simulink model "rtwdemo_preprocessor"  (Simulink 7.6)
settings: Solver=FixedStepDiscrete  StartTime=0.0  StopTime=100  FixedStep=1  RelTol=1e-3
PostLoadFcn:
  | load rtwdemo_preprocessor_data.mat
Description:
  | Code Variants Using Model Blocks
settings Model: Creator=The MathWorks Inc.
settings DataIOCC: SaveFormat=StructureWithTime
settings OptimizationCC: InlineParams=on  InlineInvariantSignals=on  StrengthReduction=on  PassReuseOutputArgsAs=Individual arguments  ZeroExternalMemoryAtStartup=off  ZeroInternalMemoryAtStartup=off  OptimizeModelRefInitCode=on  LifeSpan=1
settings DebuggingCC: MergeDetectMultiDrivingBlocksExec=error  UniqueDataStoreMsg=error  ModelReferenceSymbolNameMessage=none  StrictBusMsg=ErrorOnBusTreatedAsVector
settings HardwareCC: ProdIntDivRoundTo=Zero  ProdEndianess=LittleEndian  ProdHWDeviceType=Generic->32-bit Embedded Processor
settings ModelReferenceCC: ModelReferencePassRootInputsByReference=off
settings RTWCC: SystemTargetFile=ert.tlc  TemplateMakefile=ert_default_tmf  Description=Real-Time Workshop Embedded Coder  GenerateReport=on  RTWVerbose=off  ProcessScript=ert_make_rtw_hook  IncludeHyperlinkInReport=on  LaunchReport=on
settings CodeAppCC: IgnoreCustomStorageClasses=off  IgnoreTestpoints=on
settings ERTTargetCC: MultiwordLength=2048  GenerateSampleERTMain=on  SupportNonFinite=off  InlinedParameterPlacement=NonHierarchical  ERTCustomFileTemplate=example_file_process.tlc  ERTFilePackagingFormat=CompactWithDataFile  ConvertIfToSwitch=off

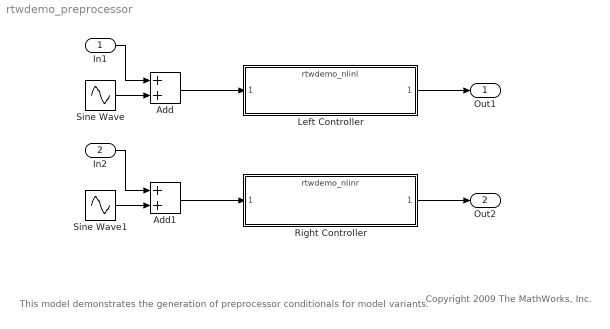
== system rtwdemo_preprocessor ==
  note: This model demonstrates the generation of
      | preprocessor conditionals for model variants.
  note: Copyright 2009 The MathWorks, Inc.
  In1 : Inport  OutDataTypeStr=double  PortDimensions=1  SampleTime=1
  In2 : Inport  Port=2  OutDataTypeStr=double  PortDimensions=1  SampleTime=1
  Add : Sum
  Add1 : Sum
  Left Controller : ModelReference  ModelNameDialog=rtwdemo_nlinl  SimulationMode=Normal  Variant=on  ModelReferenceVersion=1.22  CopyOfModelName=rtwdemo_nlinl
      settings: GeneratePreprocessorConditionals=on
  Right Controller : ModelReference  ModelNameDialog=rtwdemo_nlinr  SimulationMode=Normal  Variant=on  ModelReferenceVersion=1.22  CopyOfModelName=rtwdemo_nlinr
      settings: GeneratePreprocessorConditionals=on
  Sine Wave : Sin  SineType=Sample based  Samples=40  SampleTime=1
  Sine Wave1 : Sin  SineType=Sample based  Samples=40  SampleTime=1  Offset=20
  Out1 : Outport  OutDataTypeStr=double  PortDimensions=1  SampleTime=1
  Out2 : Outport  Port=2  OutDataTypeStr=double  PortDimensions=1  SampleTime=1
  wires:
  Add/1 -> Left Controller/1
  Left Controller/1 -> Out1/1
  Add1/1 -> Right Controller/1
  Right Controller/1 -> Out2/1
  In1/1 -> Add/1
  Sine Wave/1 -> Add/2
  In2/1 -> Add1/1
  Sine Wave1/1 -> Add1/2
